simulink model "Controller_Michiel"  (R2015b)
settings: Solver=VariableStepAuto  StartTime=0.0  StopTime=2  RelTol=1e-3
libraries: simulink x1
settings Model: Creator=MVdB  LastModifiedBy=MVdB
settings DataIOCC: ExternalInput=x,x_2  LoadExternalInput=on

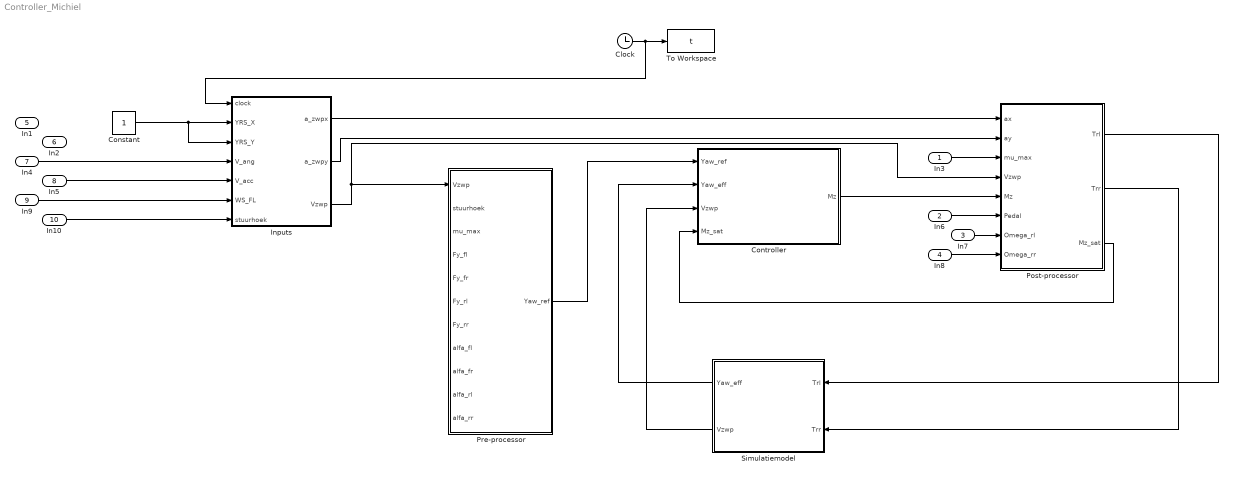
== system Controller_Michiel ==
  In3 : Inport
  In6 : Inport  Port=2
  In7 : Inport  Port=3
  In8 : Inport  Port=4
  In1 : Inport  Port=5
  In2 : Inport  Port=6
  In4 : Inport  Port=7
  In5 : Inport  Port=8
  In9 : Inport  Port=9
  In10 : Inport  Port=10
  Clock : Clock
  Constant : Constant
  Controller : Subsystem
  Inputs : MATLAB Function  TreatAsAtomicUnit=on
  Post-processor : Subsystem
  Pre-processor : MATLAB Function  TreatAsAtomicUnit=on
  Simulatiemodel : Subsystem
  To Workspace : ToWorkspace  VariableName=t  SaveFormat=Timeseries  SampleTime=-1
  wires:
  Inputs/1(a_zwpx) -> Post-processor/1(ax)
  In3/1 -> Post-processor/3(mu_max)
  Inputs/3(Vzwp) -> Post-processor/4(Vzwp), Pre-processor/1(Vzwp)
  Controller/1(Mz) -> Post-processor/5(Mz)
  In6/1 -> Post-processor/6(Pedal)
  In7/1 -> Post-processor/7(Omega_rl)
  In8/1 -> Post-processor/8(Omega_rr)
  Post-processor/1(Trl) -> Simulatiemodel/1(Trl)
  Post-processor/2(Trr) -> Simulatiemodel/2(Trr)
  Post-processor/3(Mz_sat) -> Controller/4(Mz_sat)
  Inputs/2(a_zwpy) -> Post-processor/2(ay)
  Pre-processor/1(Yaw_ref) -> Controller/1(Yaw_ref)
  Simulatiemodel/1(Yaw_eff) -> Controller/2(Yaw_eff)
  Simulatiemodel/2(Vzwp) -> Controller/3(Vzwp)
  Clock/1 -> Inputs/1(clock), To Workspace/1
  Constant/1 -> Inputs/3(YRS_Y), Inputs/2(YRS_X)
  In4/1 -> Inputs/4(V_ang)
  In5/1 -> Inputs/5(V_acc)
  In9/1 -> Inputs/6(WS_FL)
  In10/1 -> Inputs/7(stuurhoek)

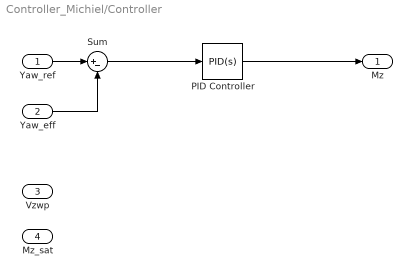
== system Controller_Michiel/Controller ==
  Yaw_ref : Inport
  Yaw_eff : Inport  Port=2
  Vzwp : Inport  Port=3
  Mz_sat : Inport  Port=4
  PID Controller : simulink/Continuous/PID Controller  Controller=PID  TimeDomain=Continuous-time  SampleTime=-1  IntegratorMethod=Forward Euler  FilterMethod=Forward Euler  Form=Parallel  UseFilter=on  ControllerParametersSource=internal  P=1  I=1  D=0  N=100  InitialConditionSource=internal  InitialConditionForIntegrator=0  InitialConditionForFilter=0  ExternalReset=none  LimitOutput=off  UpperSaturationLimit=inf  LowerSaturationLimit=-inf  LinearizeAsGain=on  AntiWindupMode=none  Kb=1  TrackingMode=off  Kt=1  PParamMin=[]  PParamMax=[]  IParamMin=[]  IParamMax=[]  DParamMin=[]  DParamMax=[]  NParamMin=[]  NParamMax=[]  KbParamMin=[]  KbParamMax=[]  KtParamMin=[]  KtParamMax=[]  POutMin=[]  POutMax=[]  IOutMin=[]  IOutMax=[]  DOutMin=[]  DOutMax=[]  NOutMin=[]  NOutMax=[]  KbOutMin=[]  KbOutMax=[]  KtOutMin=[]  KtOutMax=[]  IntegratorOutMin=[]  IntegratorOutMax=[]  FilterOutMin=[]  FilterOutMax=[]  SumOutMin=[]  SumOutMax=[]  SumI1OutMin=[]  SumI1OutMax=[]  SumI2OutMin=[]  SumI2OutMax=[]  SumI3OutMin=[]  SumI3OutMax=[]  SumDOutMin=[]  SumDOutMax=[]  SaturationOutMin=[]  SaturationOutMax=[]  IntegratorContinuousStateAttributes=''  IntegratorStateMustResolveToSignalObject=off  IntegratorRTWStateStorageClass=Auto  FilterContinuousStateAttributes=''  FilterStateMustResolveToSignalObject=off  FilterRTWStateStorageClass=Auto  DifferentiatorICPrevScaledInput=0  DifferentiatorOutMin=[]  DifferentiatorOutMax=[]
  Sum : Sum  Inputs=|+-
  Mz : Outport
  wires:
  Yaw_ref/1 -> Sum/1
  Yaw_eff/1 -> Sum/2
  Sum/1 -> PID Controller/1
  PID Controller/1 -> Mz/1

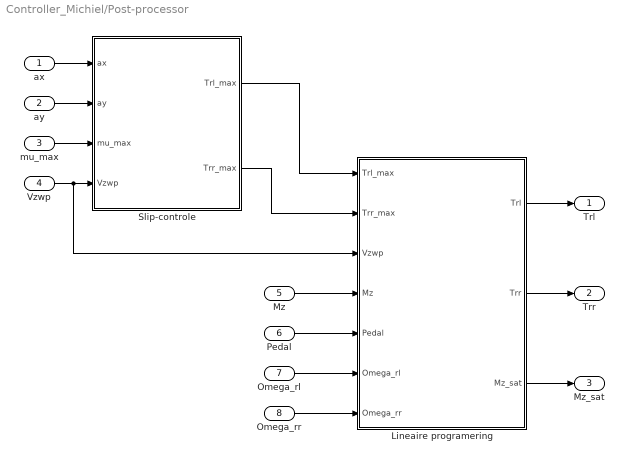
== system Controller_Michiel/Post-processor ==
  ax : Inport
  ay : Inport  Port=2
  mu_max : Inport  Port=3
  Vzwp : Inport  Port=4
  Mz : Inport  Port=5
  Pedal : Inport  Port=6
  Omega_rl : Inport  Port=7
  Omega_rr : Inport  Port=8
  Lineaire programering : MATLAB Function  TreatAsAtomicUnit=on
  "Slip-controle " : MATLAB Function  TreatAsAtomicUnit=on
  Trl : Outport
  Trr : Outport  Port=2
  Mz_sat : Outport  Port=3
  wires:
  "Slip-controle "/2(Trr_max) -> Lineaire programering/2(Trr_max)
  "Slip-controle "/1(Trl_max) -> Lineaire programering/1(Trl_max)
  ay/1 -> "Slip-controle "/2(ay)
  ax/1 -> "Slip-controle "/1(ax)
  Lineaire programering/3(Mz_sat) -> Mz_sat/1
  Lineaire programering/2(Trr) -> Trr/1
  Lineaire programering/1(Trl) -> Trl/1
  Vzwp/1 -> Lineaire programering/3(Vzwp), "Slip-controle "/4(Vzwp)
  mu_max/1 -> "Slip-controle "/3(mu_max)
  Mz/1 -> Lineaire programering/4(Mz)
  Omega_rl/1 -> Lineaire programering/6(Omega_rl)
  Pedal/1 -> Lineaire programering/5(Pedal)
  Omega_rr/1 -> Lineaire programering/7(Omega_rr)

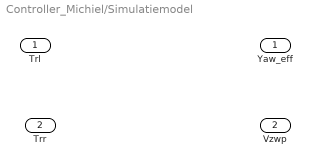
== system Controller_Michiel/Simulatiemodel ==
  Trl : Inport
  Trr : Inport  Port=2
  Yaw_eff : Outport
  Vzwp : Outport  Port=2

== matlab function Controller_Michiel/Post-processor/Lineaire programering ==
  data: Trl_max input; Trl output; Trr_max input; Vzwp input; Mz input; Pedal input; Omega_rl input; Omega_rr input; Trr output; Mz_sat output
function [Trl,Trr,Mz_sat] = Lineaire_programmering(Trl_max,Trr_max,Vzwp,Mz,Pedal,Omega_rl,Omega_rr)
%Deze blok staat in voor het berekenen van de te leveren torque per wiel
%aan de hand van twee lineaire doelen. Het eerste doel is het netto moment
%rond het zwaartepunt optimaliseren. Het tweede doel is de torque die wordt
%overgedragen op het wegdek optimaliseren.

%%
M       =265;               
L       =1.525;             
Lf      =0.780;             
Lr      =0.745;             
Tf      =1.200;             
Tr      =1.200;             
g       =9.81;              
Ksf     =12153;             
Ksr     =14563;             
Krf_a	=183.26;            
Krr_a	=325.31;            
Kwf     =0;                 
Kwr     =0;                 
Hrcf	=0.032;             
Hrcr	=0.041;             
Hurcf	=0;                 
Hurcr	=0;                 
H       =0.2735;            
D       =0.2369;            
Rm      =576.35;            
Reff	=0.2325;            
Gr      =10.32;             
Sr      =0.600;             
Tmax	=77;              
Cte     =0;                 
ax      =0;                 
ay      =0;                 
Mu_f    =8.5;               
Mu_r    =8.5;               
R1      =0;                 
R2      =0;                 
R4_x    =0;                 
R4_y    =0;                 
Vzwp    =0;                 
mu_max  =0.9;
Pmax    =150000; 


coder.extrinsic('eval','num2str','linprog','mxgetdata');

Ttot    = 0;

%%
%voorbereidende berekeningen
Omega = abs((Omega_rl + Omega_rr) / 2);

Tmax = min(Tmax,(Pmax/Omega)) ;

TV_control = (Mz*Reff)/(2*Sr*Gr) ;

%%
%Gevraagd Moment
TV_max_1 = min(40,((Trl_max+Trr_max)/2));

maximum1 = 2*max(-TV_max_1,min(TV_max_1,TV_control));

%Maken van variabelen
variables1 = {'Trr_1','Trl_1','e','maxi'};
N = length(variables1); 
% create variables for indexing 
for v = 1:N 
   eval([variables1{v},' = ', num2str(v),';']); 
end

%Ondergrenzen bepalen
lb = zeros(size(variables1));
lb([1 2 3]) = [-40,-40,0];

%Bovengrenzen bepalen
ub = Inf(size(variables1));
ub([1 2]) = [40,40];

%Ongelijkheden
A = zeros(2,4); b = zeros(1,4);
A(1,1) = 1; A(1,2) = 1; b(1) = Tmax;
A(2,4) = 1; b(2) = maximum1;

%Gelijkheden
Aeq = zeros(1,4); beq = zeros(1,1);
Aeq(1,[1 2 3 4]) = [1,-1,1,-1];

%Te optimaliseren kostenfunctie
f = zeros(size(variables1));
f([1 2 3]) = [-1 -1 -1];

%Optimalisatie
x = linprog(f,A,b,Aeq,beq,lb,ub);



%%
%Gevraagde torque
mini = [40 (Trl_max-(Ttot/2)) (Trr_max+(Ttot/2))];
TV_max_2 = max(0,min(mini));
maximum2 = 2*max(-TV_max_2,min(TV_max_2,TV_control));

%Maken van variabelen
variables2 = {'Trr_2','Trl_2','maxi'};
N = length(variables2); 
% create variables for indexing 
for v = 1:N 
   eval([variables2{v},' = ', num2str(v),';']); 
end

%Ondergrenzen bepalen
lb_2 = zeros(size(variables2));
lb_2([1 2]) = [-40,-40];

%Bovengrenzen bepalen
ub_2 = Inf(size(variables2));
ub_2([1 2]) = [40,40];

%Ongelijkheden
A_2 = zeros(2,3); b_2 = zeros(1,3);
A_2(1,1) = 1; A_2(1,2) = 1; b_2(1) = Tmax;
A_2(2,3) = 1; b_2(2) = maximum2;

%Gelijkheden
Aeq_2 = zeros(1,3); beq_2 = zeros(1,1);
Aeq_2(1,[1 2 3]) = [1,-1,-1];

%Te optimaliseren kostenfunctie
f_2 = zeros(size(variables2));
f_2([1 2]) = [-1 -1];

%Optimalisatie
x_2 = linprog(f_2,A_2,b_2,Aeq_2,beq_2,lb_2,ub_2);


%%
%Effectieve torques naar motordrives
Trl_1 = x.x(2);
Trl_2 = x_2.x_2(2);
Trr_1 = x.x(1);
Trr_2 = x_2.x_2(1);

Trl = Trl_1*Cte + Trl_2*(1-Cte);
Trr = Trr_1*Cte + Trr_2*(1-Cte);

== matlab function Controller_Michiel/Post-processor/Slip-controle  ==
  data: ax input; ay input; mu_max input; Trl_max output; Vzwp input; Trr_max output
function [Trl_max,Trr_max] = Slip_controle(ax,ay,mu_max,Vzwp)
% Berekening van de maximale torques die men kan toepassen op de wielen
% door berekening van de normaalkrachten op de wielen.

%load('parameters.mat');

M       =265;               
L       =1.525;             
Lf      =0.780;             
Lr      =0.745;             
Tf      =1.200;             
Tr      =1.200;             
g       =9.81;              
Ksf     =12153;             
Ksr     =14563;             
Krf_a	=183.26;            
Krr_a	=325.31;            
Kwf     =0;                 
Kwr     =0;                 
Hrcf	=0.032;             
Hrcr	=0.041;             
Hurcf	=0;                 
Hurcr	=0;                 
H       =0.2735;            
D       =0.2369;            
Rm      =576.35;            
Reff	=0.2325;            
Gr      =10.32;             
Sr      =0.600;             
Tmax	=38.5;              
Cte     =0;                 
ax      =0;                 
ay      =0;                 
Mu_f    =8.5;               
Mu_r    =8.5;               
R1      =0;                 
R2      =0;                 
R4_x    =0;                 
R4_y    =0;                 
Vzwp    =0;                 
mu_max  =0.9;

%Wielbelastingen

%Statische wielbelasting
Ws_fl = (Lf/(2*L))*M*g;
Ws_fr = Ws_fl;
Ws_rl = (Lr/(2*L))*M*g;
Ws_rr = Ws_rl;

Ws_f = Ws_fl + Ws_fr;
Ws_r = Ws_rl + Ws_rr;

%Laterale wielbelasting (door rollen van de wagen)
FfsM = (Ksf*M*ay*D)/(Tf*(Ksf+Ksr-(M*g*D)));   %Kracht door rolmoment
FrsM = (Ksr*M*ay*D)/(Tr*(Ksf+Ksr-(M*g*D)));

FfsF = (Ws_f*ay*Hrcf)/Tf;                    %Kracht door afgeveerde massa
FrsF = (Ws_r*ay*Hrcr)/Tr;

FfuF = (Mu_f*ay*Hurcf)/Tf;                   %Kracht door onafgeveerde massa
FruF = (Mu_r*ay*Hurcr)/Tr;

Ff = FfsM + FfsF + FfuF;                    %Totale gewichtsverplaatsing
Fr = FrsM + FrsF + FruF;

Wy_fl = Ff/2;                               %Kracht per wiel
Wy_fr = -Wy_fl;
Wy_rl = Fr/2;
Wy_rr = -Wy_rl;

%Longitudinale wielbelasting
Wx_fl = (-H/(2*L))*M*ax;
Wx_fr = Wx_fl;
Wx_rl = (H/(2*L))*M*ax;
Wx_rr = Wx_rl;

%Aerodynamische wielbelasting
LF = -0.0237*(Vzwp)^2 + 0.0958*Vzwp;                %Nog na te kijken
LR = -0.0237*(Vzwp)^2 + 0.0958*Vzwp;                %Nog na te kijken

Wa_fl = (-LF/(2*L));  %+((Krf/(Krf+Krr))*(Rm/Tf));      %is er hier 2x rolmoment??? (zie lateraal)
Wa_fr = (-LF/(2*L));  %-((Krf/(Krf+Krr))*(Rm/Tf));
Wa_rl = (-LR/(2*L));  %+((Krr/(Krf+Krr))*(Rm/Tr));
Wa_rr = (-LR/(2*L));  %-((Krr/(Krf+Krr))*(Rm/Tr));

%anti-roll bar wielbelasting
Wab_fl = (Krf_a/((Krf_a+((Kwf*(Tf)^2)/2))*Wy_fl));
Wab_fr = -Wab_fl;
Wab_rl = (Krr_a/((Krr_a+((Kwr*(Tr)^2)/2))*Wy_rl));
Wab_rr = -Wab_rl;

%Totale belasting per wiel
Wfl = Ws_fl + Wy_fl + Wx_fl + Wa_fl + Wab_fl;   %Ongebruikt, kan later eventueel gebruikt worden voor 4WD
Wfr = Ws_fr + Wy_fr + Wx_fr + Wa_fr + Wab_fr;   %^ Idem
Wrl = Ws_rl + Wy_rl + Wx_rl + Wa_rl + Wab_rl;
Wrr = Ws_rr + Wy_rr + Wx_rr + Wa_rr + Wab_rr;



%%Omrekening naar torques

%Wrijvingscirkels
Fx_rl = sqrt((Wrl^2*mu_max^2)-(Wrl^2*ay^2));
Fx_rr = sqrt((Wrr^2*mu_max^2)-(Wrr^2*ay^2));

%Maximum torques
Trl_max = Fx_rl*Reff;
Trr_max = Fx_rr*Reff;

== matlab function Controller_Michiel/Pre-processor ==
  data: Yaw_ref output; Vzwp input; stuurhoek input; mu_max input; Fy_fl input; Fy_fr input; Fy_rl input; Fy_rr input; alfa_fl input; alfa_fr input; alfa_rl input; alfa_rr input
function Yaw_ref  = pre_processor(Vzwp,stuurhoek,mu_max,Fy_fl,Fy_fr,Fy_rl,Fy_rr,alfa_fl,alfa_fr,alfa_rl,alfa_rr)
%De pre-processor berekend de gewenste yaw rate door het minimum te nemen
%van de ideale en de maximale yaw rate waarde.


M       =265;               
L       =1.525;             
Lf      =0.780;             
Lr      =0.745;             
Tf      =1.200;             
Tr      =1.200;             
g       =9.81;              
Ksf     =12153;             
Ksr     =14563;             
Krf_a	=183.26;            
Krr_a	=325.31;            
Kwf     =0;                 
Kwr     =0;                 
Hrcf	=0.032;             
Hrcr	=0.041;             
Hurcf	=0;                 
Hurcr	=0;                 
H       =0.2735;            
D       =0.2369;            
Rm      =576.35;            
Reff	=0.2325;            
Gr      =10.32;             
Sr      =0.600;             
Tmax	=38.5;              
Cte     =0;                 
ax      =0;                 
ay      =0;                 
Mu_f    =8.5;               
Mu_r    =8.5;               
R1      =0;                 
R2      =0;                 
R4_x    =0;                 
R4_y    =0;                 
Vzwp    =0;                 
mu_max  =0.9;

X = [];
%Berekening massa's
Mf = M*(Lr/L);
Mr = M*(Lf/L);

%Berekening Cornering stiffness
C_fl = (Fy_fl/alfa_fl);
C_fr = (Fy_fr/alfa_fr);
C_rl = (Fy_rl/alfa_rl);
C_rr = (Fy_rr/alfa_rr);

%Gemiddelde van de cornering stiffness vooraan en achteraan nemen
 Cf = ((C_fl + C_fr)/ 2);
 Cr = ((C_rl + C_rr)/ 2);
%Berekening van de onderstuur factor.
Ku = ((Mf/Cf)-(Mr/Cr));

%Berekening van de ideale yaw rate.
Yaw_id = ((Vzwp*stuurhoek)/((Lf+Lr)+Ku*(Vzwp)^2));
X = [X Yaw_id];
% berekening van de sliphoek beita
beta = atan(Lf * tan(stuurhoek)/ (Lf+Lr)) ;

%Berekening van de maximale yaw rate.
Yaw_max = ((mu_max*g)/(Vzwp*cos(beta)))-Vzwp*diff(beta)*cos(beta);
X = [X Yaw_max];
%Minimale yaw rate.
M = min(X);
Yaw_ref = M;

== matlab function Controller_Michiel/Inputs ==
  data: clock input; YRS_X input; YRS_Y input; V_ang input; V_acc input; WS_FL input; a_zwpx output; a_zwpy output; stuurhoek input; Vzwp output
function [a_zwpx,a_zwpy,Vzwp]= Inputs(clock,YRS_X,YRS_Y,V_ang,V_acc,WS_FL,stuurhoek)
% hier zullen de inputs verwerkt worden die nodig zijn voor de 
    % aansturing van het controle algortihme.
    %
    % YRS is de versnelling die gemeten word door de yaw-rate sensor
    % V_ang is de hoeksnelheid       
    % V_acc is de hoekversnelling
    
R1 = 0;
R2 = 0.100;
YRS_X = 2;
YRS_Y = 2;
V_acc = 1;
V_ang = 1;
t = 1;
Reff = 0.2325;
C = 0;
R4_x = 0.100;
R4_y = 0.050;


% berekening van de versnelling van het zwaartepunt in de x-richting
a_zwpx = YRS_X + (V_acc *R2) + V_ang*(V_ang*R1);

% versnelling in de y-richting
a_zwpy = YRS_Y + (V_acc *R1) + V_ang*(V_ang*R2);

% Totale versnelling van het zwaartepunt
a_zwp = sqrt ((a_zwpx^2) + (a_zwpy^2)); 
    
% De snelheid van het zwaartepunt
if clock == 0                           % beginconditie integratieterm = 0 
    C = 0;
end
    
Vzwpacc = a_zwp*clock + C;              % C is de beginsnelheid
C = Vzwpacc;
  
    % De snelheid op bassis van de wielspeed sensoren 
    % V_FL is de snelheid van het linker voorwiel, WS_FL is de hoeksnelheid van
    % dit wiel en R3 is de banden straal

V_FL = WS_FL * Reff ;
v_zwpwiel = V_FL *cos(stuurhoek)+ V_FL * sin (stuurhoek) + V_ang * (R4_x - R4_y);

 % vergelijken van deze twee snelheden
 
 if (v_zwpwiel- Vzwpacc)> -0.05   && (v_zwpwiel- Vzwpacc)< 0.05       
        V = v_zwpwiel;                  % wagen slipt niet
 else
        V = Vzwpacc;                    % wagen slipt              
 
 end
 
 Vzwp = V;
